simulink model "Lorenzo_comparison_simulation"  (R2023b)
settings: Solver=ode5  StartTime=0.0  StopTime=8  FixedStep=0.00005  RelTol=1e-3
settings Model: Creator=amaiani  LastModifiedBy=amaiani

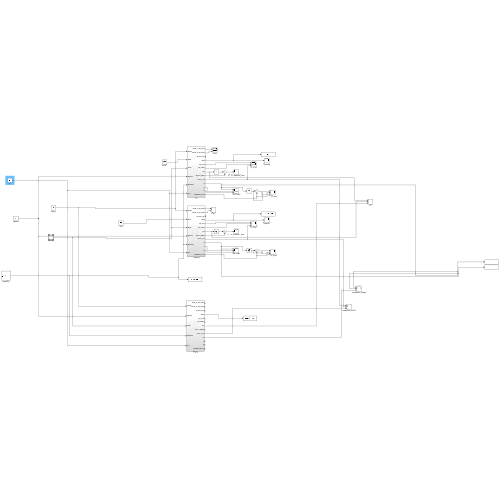
[thumbnail: Simulink's stored preview of the top-level diagram]
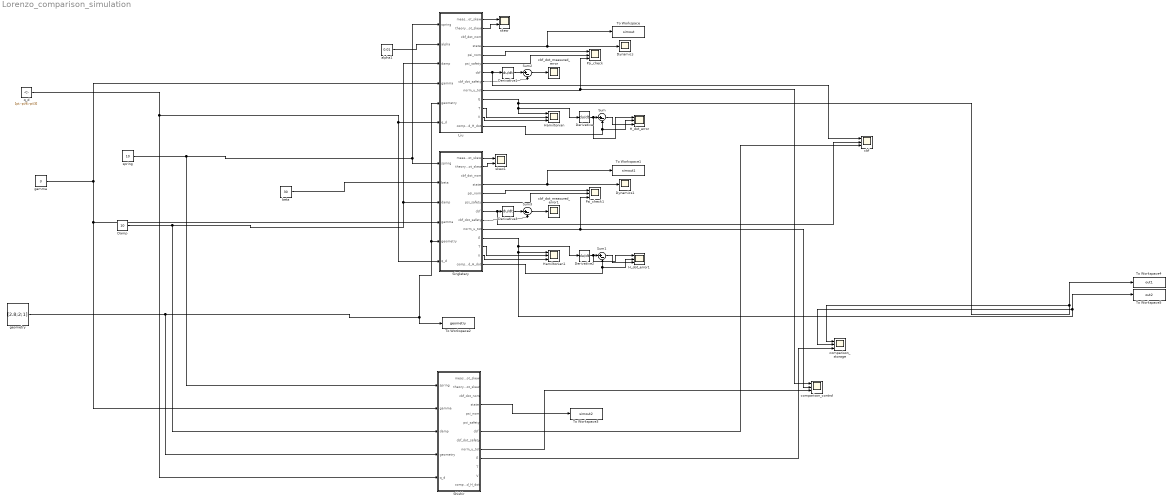
== system Lorenzo_comparison_simulation ==
  Damp : Constant  Value=10
  Derivative{,1..3} (4 alike) : Derivative
  Dynamics : Scope
  Dynamics1 : Scope
  H_dot_error : Scope  NumInputPorts=3
  H_dot_error1 : Scope  NumInputPorts=3
  Hamiltonian : Scope  NumInputPorts=3
  Hamiltonian1 : Scope  NumInputPorts=3
  Liu : Subsystem
  Psi_check : Scope  NumInputPorts=3
  Psi_check1 : Scope  NumInputPorts=3
  Shishir : Subsystem
  Singletary : Subsystem
  Sum{,1..3} (4 alike) : Sum  Inputs=|+-
  To Workspace : ToWorkspace  VariableName=simout  SampleTime=-1
  To Workspace1 : ToWorkspace  VariableName=simout1  SampleTime=-1
  To Workspace2 : ToWorkspace  VariableName=geometry  SampleTime=-1
  To Workspace3 : ToWorkspace  VariableName=simout2  SampleTime=-1
  To Workspace4 : ToWorkspace  VariableName=out1  SampleTime=-1
  To Workspace5 : ToWorkspace  VariableName=out2  SampleTime=-1
  alpha1 : Constant  Value=0.01
  beta : Constant  Value=30
  cbf : Scope  NumInputPorts=3
  cbf_dot_measured_error : Scope
  cbf_dot_measured_error1 : Scope
  comparison_control : Scope  NumInputPorts=3
  comparison_storage : Scope  NumInputPorts=3
  gamma : Constant  Value=3
  geometry : Constant  Value=[2.8;2;1]
  q_d : Constant  Value=[pi;-pi/6;-pi/3]
  skew : Scope  NumInputPorts=2
  skew1 : Scope  NumInputPorts=2
  spring : Constant  Value=10
  wires:
  Liu/10(E) -> To Workspace4/1, comparison_storage/1, Derivative/1, Hamiltonian/1
  Liu/1(meas_m_dot_skew) -> skew/1
  Liu/2(theory_m_dot_skew) -> skew/2
  Liu/13(computed_H_dot) -> H_dot_error/2, Sum/2
  Liu/7(cbf) -> cbf/1, Derivative1/1
  Derivative1/1 -> Sum2/1
  Sum2/1 -> cbf_dot_measured_error/1
  Liu/8(cbf_dot_safety) -> Sum2/2
  Liu/11(T) -> Hamiltonian/2
  Liu/12(V) -> Hamiltonian/3
  gamma/1 -> Singletary/4(gamma), Shishir/2(gamma), Liu/4(gamma)
  Derivative/1 -> H_dot_error/1, Sum/1
  Sum/1 -> H_dot_error/3
  Liu/9(norm_u_tot) -> comparison_control/1, Psi_check/3
  Liu/6(psi_safety) -> Psi_check/2
  Liu/5(psi_nom) -> Psi_check/1
  Liu/4(state) -> Dynamics/1, To Workspace/1
  Singletary/2(theory_m_dot_skew) -> skew1/2
  Sum3/1 -> cbf_dot_measured_error1/1
  Singletary/8(cbf_dot_safety) -> Sum3/2
  Singletary/11(T) -> Hamiltonian1/2
  Derivative3/1 -> Sum3/1
  Singletary/12(V) -> Hamiltonian1/3
  Singletary/4(state) -> Dynamics1/1, To Workspace1/1
  Singletary/6(psi_safety) -> Psi_check1/2
  Singletary/1(meas_m_dot_skew) -> skew1/1
  Singletary/5(psi_nom) -> Psi_check1/1
  Derivative2/1 -> H_dot_error1/1, Sum1/1
  Singletary/13(computed_H_dot) -> H_dot_error1/2, Sum1/2
  Singletary/9(norm_u_tot) -> comparison_control/2, Psi_check1/3
  Sum1/1 -> H_dot_error1/3
  Singletary/7(cbf) -> cbf/2, Derivative3/1
  geometry/1 -> Shishir/4(geometry), Liu/5(geometry), Singletary/5(geometry), To Workspace2/1
  alpha1/1 -> Liu/2(alpha)
  Damp/1 -> Shishir/3(damp), Singletary/3(damp), Liu/3(damp)
  spring/1 -> Shishir/1(spring), Singletary/1(spring), Liu/1(spring)
  beta/1 -> Singletary/2(beta)
  Singletary/10(E) -> To Workspace5/1, comparison_storage/2, Hamiltonian1/1, Derivative2/1
  Shishir/7(cbf) -> cbf/3
  Shishir/10(E) -> comparison_storage/3
  Shishir/9(norm_u_tot) -> comparison_control/3
  q_d/1 -> Shishir/5(q_d), Liu/6(q_d), Singletary/6(q_d)
  Shishir/4(state) -> To Workspace3/1

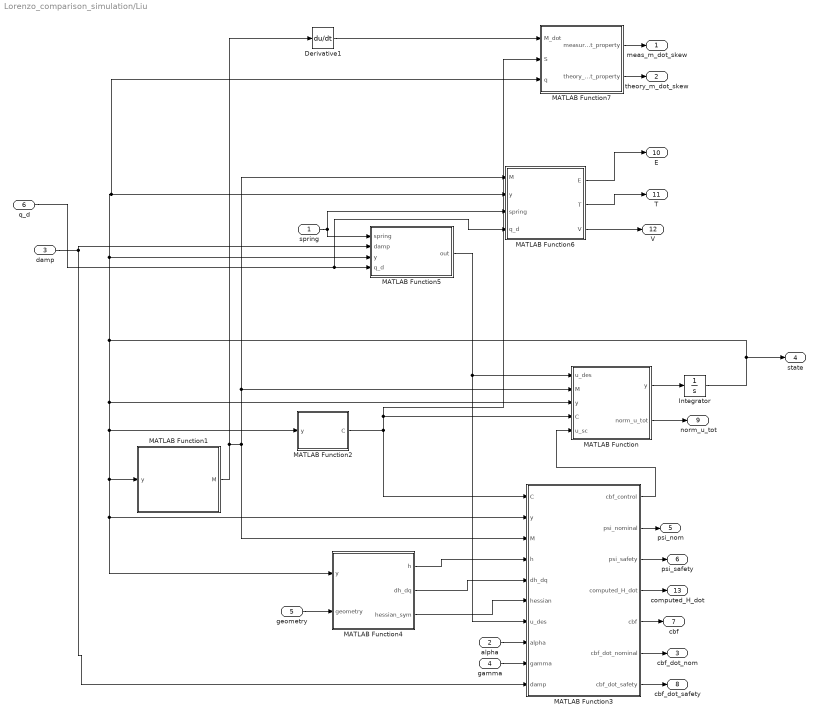
== system Lorenzo_comparison_simulation/Liu ==
  spring : Inport
  alpha : Inport  Port=2
  damp : Inport  Port=3
  gamma : Inport  Port=4
  geometry : Inport  Port=5
  q_d : Inport  Port=6
  Derivative1 : Derivative
  Integrator : Integrator  InitialCondition=[0;0;0;0;0;0]
  MATLAB Function : MATLAB Function  TreatAsAtomicUnit=on
  MATLAB Function1 : MATLAB Function  StartFcn=|  TreatAsAtomicUnit=on
      | % Define numerical values for the parameters
      | xc = 2.5;
      | yc = 2;
      | r = 1;
      | gamma = 2;
      | alpha = 20;
      | 
      | 
      | m1 = 1;
      | m2 = 1;
      | m3 = 1;
      | 
      | 
      | l1 = 1;
      | l2 = 1;
      | l3 = 1;
  MATLAB Function2 : MATLAB Function  StartFcn=|  TreatAsAtomicUnit=on
      | % Define numerical values for the parameters
      | xc = 2.5;
      | yc = 2;
      | r = 1;
      | gamma = 2;
      | alpha = 20;
      | 
      | 
      | m1 = 1;
      | m2 = 1;
      | m3 = 1;
      | 
      | 
      | l1 = 1;
      | l2 = 1;
      | l3 = 1;
  MATLAB Function3 : MATLAB Function  TreatAsAtomicUnit=on
  MATLAB Function4 : MATLAB Function  TreatAsAtomicUnit=on
  MATLAB Function5 : MATLAB Function  TreatAsAtomicUnit=on
  MATLAB Function6 : MATLAB Function  TreatAsAtomicUnit=on
  MATLAB Function7 : MATLAB Function  StartFcn=|  TreatAsAtomicUnit=on
      | % Define numerical values for the parameters
      | xc = 2.5;
      | yc = 2;
      | r = 1;
      | gamma = 2;
      | alpha = 20;
      | 
      | 
      | m1 = 1;
      | m2 = 1;
      | m3 = 1;
      | 
      | 
      | l1 = 1;
      | l2 = 1;
      | l3 = 1;
  meas_m_dot_skew : Outport
  theory_m_dot_skew : Outport  Port=2
  cbf_dot_nom : Outport  Port=3
  state : Outport  Port=4
  psi_nom : Outport  Port=5
  psi_safety : Outport  Port=6
  cbf : Outport  Port=7
  cbf_dot_safety : Outport  Port=8
  norm_u_tot : Outport  Port=9
  E : Outport  Port=10
  T : Outport  Port=11
  V : Outport  Port=12
  computed_H_dot : Outport  Port=13
  wires:
  MATLAB Function3/7(cbf_dot_safety) -> cbf_dot_safety/1
  MATLAB Function3/2(psi_nominal) -> psi_nom/1
  MATLAB Function3/5(cbf) -> cbf/1
  MATLAB Function/2(norm_u_tot) -> norm_u_tot/1
  MATLAB Function4/3(hessian_sym) -> MATLAB Function3/6(hessian)
  MATLAB Function1/1(M) -> Derivative1/1, MATLAB Function6/1(M), MATLAB Function/2(M), MATLAB Function3/3(M)
  MATLAB Function4/2(dh_dq) -> MATLAB Function3/5(dh_dq)
  MATLAB Function7/1(measured_m_dot_property) -> meas_m_dot_skew/1
  alpha/1 -> MATLAB Function3/8(alpha)
  MATLAB Function6/1(E) -> E/1
  MATLAB Function3/3(psi_safety) -> psi_safety/1
  MATLAB Function7/2(theory_m_dot_property) -> theory_m_dot_skew/1
  MATLAB Function3/4(computed_H_dot) -> computed_H_dot/1
  Derivative1/1 -> MATLAB Function7/1(M_dot)
  q_d/1 -> MATLAB Function6/4(q_d), MATLAB Function5/4(q_d)
  MATLAB Function3/6(cbf_dot_nominal) -> cbf_dot_nom/1
  MATLAB Function/1(y) -> Integrator/1
  MATLAB Function3/1(cbf_control) -> MATLAB Function/5(u_sc)
  MATLAB Function2/1(C) -> MATLAB Function/4(C), MATLAB Function7/2(S), MATLAB Function3/1(C)
  MATLAB Function4/1(h) -> MATLAB Function3/4(h)
  spring/1 -> MATLAB Function6/3(spring), MATLAB Function5/1(spring)
  MATLAB Function5/1(out) -> MATLAB Function3/7(u_des), MATLAB Function/1(u_des)
  Integrator/1 -> MATLAB Function7/3(q), MATLAB Function6/2(y), MATLAB Function5/3(y), MATLAB Function4/1(y), MATLAB Function3/2(y), MATLAB Function1/1(y), MATLAB Function2/1(y), MATLAB Function/3("y "), state/1
  damp/1 -> MATLAB Function3/10(damp), MATLAB Function5/2(damp)
  MATLAB Function6/2(T) -> T/1
  MATLAB Function6/3(V) -> V/1
  gamma/1 -> MATLAB Function3/9(gamma)
  geometry/1 -> MATLAB Function4/2(geometry)

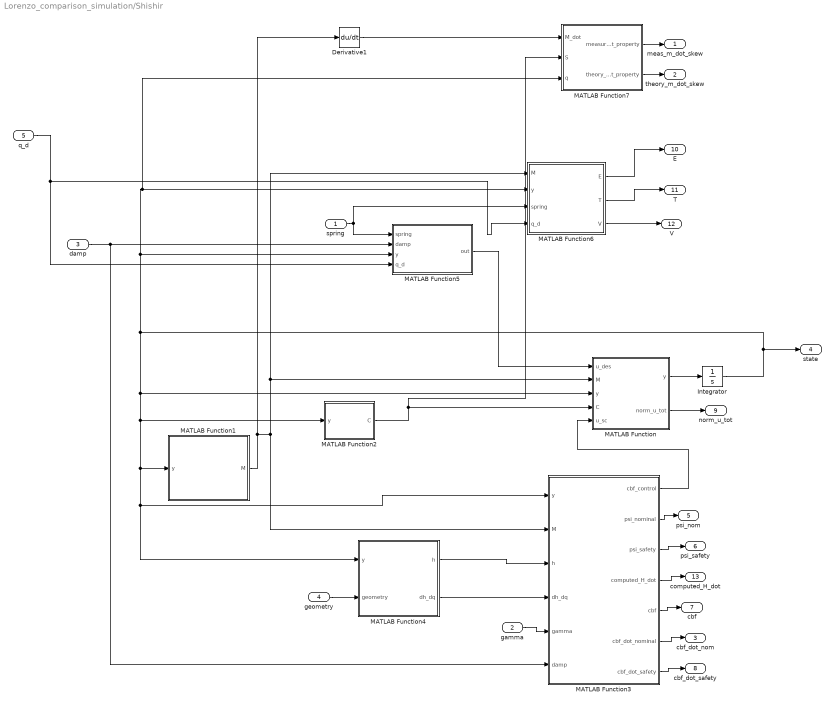
== system Lorenzo_comparison_simulation/Shishir ==
  spring : Inport
  gamma : Inport  Port=2
  damp : Inport  Port=3
  geometry : Inport  Port=4
  q_d : Inport  Port=5
  Derivative1 : Derivative
  Integrator : Integrator  InitialCondition=[0;0;0;0;0;0]
  MATLAB Function : MATLAB Function  TreatAsAtomicUnit=on
  MATLAB Function1 : MATLAB Function  StartFcn=|  TreatAsAtomicUnit=on
      | % Define numerical values for the parameters
      | xc = 2.5;
      | yc = 2;
      | r = 1;
      | gamma = 2;
      | alpha = 20;
      | 
      | 
      | m1 = 1;
      | m2 = 1;
      | m3 = 1;
      | 
      | 
      | l1 = 1;
      | l2 = 1;
      | l3 = 1;
  MATLAB Function2 : MATLAB Function  StartFcn=|  TreatAsAtomicUnit=on
      | % Define numerical values for the parameters
      | xc = 2.5;
      | yc = 2;
      | r = 1;
      | gamma = 2;
      | alpha = 20;
      | 
      | 
      | m1 = 1;
      | m2 = 1;
      | m3 = 1;
      | 
      | 
      | l1 = 1;
      | l2 = 1;
      | l3 = 1;
  MATLAB Function3 : MATLAB Function  TreatAsAtomicUnit=on
  MATLAB Function4 : MATLAB Function  TreatAsAtomicUnit=on
  MATLAB Function5 : MATLAB Function  TreatAsAtomicUnit=on
  MATLAB Function6 : MATLAB Function  TreatAsAtomicUnit=on
  MATLAB Function7 : MATLAB Function  StartFcn=|  TreatAsAtomicUnit=on
      | % Define numerical values for the parameters
      | xc = 2.5;
      | yc = 2;
      | r = 1;
      | gamma = 2;
      | alpha = 20;
      | 
      | 
      | m1 = 1;
      | m2 = 1;
      | m3 = 1;
      | 
      | 
      | l1 = 1;
      | l2 = 1;
      | l3 = 1;
  meas_m_dot_skew : Outport
  theory_m_dot_skew : Outport  Port=2
  cbf_dot_nom : Outport  Port=3
  state : Outport  Port=4
  psi_nom : Outport  Port=5
  psi_safety : Outport  Port=6
  cbf : Outport  Port=7
  cbf_dot_safety : Outport  Port=8
  norm_u_tot : Outport  Port=9
  E : Outport  Port=10
  T : Outport  Port=11
  V : Outport  Port=12
  computed_H_dot : Outport  Port=13
  wires:
  MATLAB Function3/7(cbf_dot_safety) -> cbf_dot_safety/1
  MATLAB Function3/2(psi_nominal) -> psi_nom/1
  MATLAB Function3/5(cbf) -> cbf/1
  MATLAB Function/2(norm_u_tot) -> norm_u_tot/1
  MATLAB Function1/1(M) -> Derivative1/1, MATLAB Function6/1(M), MATLAB Function/2(M), MATLAB Function3/2(M)
  MATLAB Function4/2(dh_dq) -> MATLAB Function3/4(dh_dq)
  MATLAB Function7/1(measured_m_dot_property) -> meas_m_dot_skew/1
  gamma/1 -> MATLAB Function3/5(gamma)
  MATLAB Function6/1(E) -> E/1
  MATLAB Function3/3(psi_safety) -> psi_safety/1
  MATLAB Function7/2(theory_m_dot_property) -> theory_m_dot_skew/1
  MATLAB Function3/4(computed_H_dot) -> computed_H_dot/1
  Derivative1/1 -> MATLAB Function7/1(M_dot)
  q_d/1 -> MATLAB Function6/4(q_d), MATLAB Function5/4(q_d)
  MATLAB Function3/6(cbf_dot_nominal) -> cbf_dot_nom/1
  MATLAB Function/1(y) -> Integrator/1
  MATLAB Function3/1(cbf_control) -> MATLAB Function/5(u_sc)
  MATLAB Function2/1(C) -> MATLAB Function/4(C), MATLAB Function7/2(S)
  MATLAB Function4/1(h) -> MATLAB Function3/3(h)
  spring/1 -> MATLAB Function6/3(spring), MATLAB Function5/1(spring)
  MATLAB Function5/1(out) -> MATLAB Function/1(u_des)
  Integrator/1 -> MATLAB Function7/3(q), MATLAB Function6/2(y), MATLAB Function5/3(y), MATLAB Function4/1(y), MATLAB Function3/1(y), MATLAB Function1/1(y), MATLAB Function2/1(y), MATLAB Function/3("y "), state/1
  damp/1 -> MATLAB Function3/6(damp), MATLAB Function5/2(damp)
  MATLAB Function6/2(T) -> T/1
  MATLAB Function6/3(V) -> V/1
  geometry/1 -> MATLAB Function4/2(geometry)

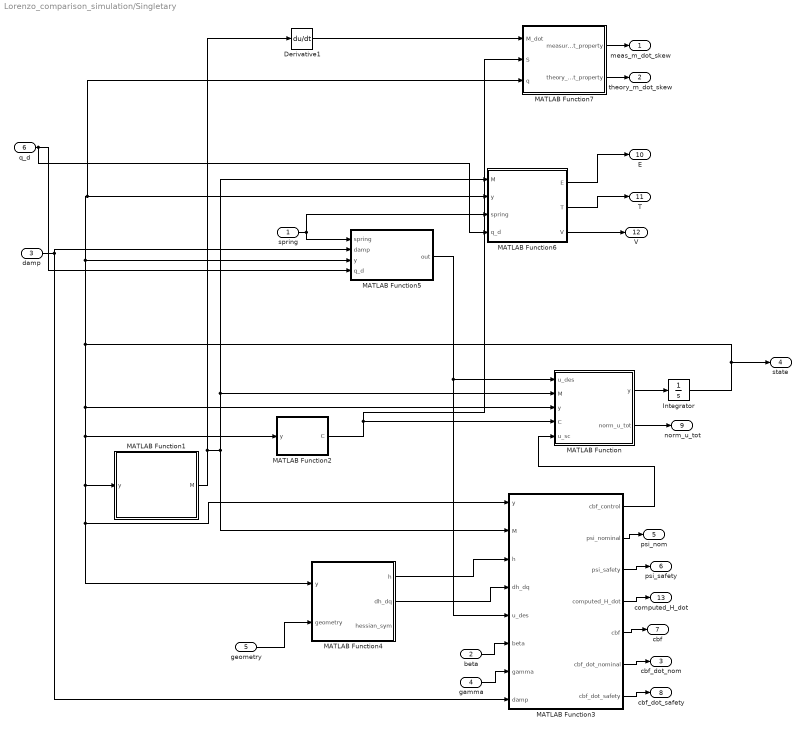
== system Lorenzo_comparison_simulation/Singletary ==
  spring : Inport
  beta : Inport  Port=2
  damp : Inport  Port=3
  gamma : Inport  Port=4
  geometry : Inport  Port=5
  q_d : Inport  Port=6
  Derivative1 : Derivative
  Integrator : Integrator  InitialCondition=[0;0;0;0;0;0]
  MATLAB Function : MATLAB Function  TreatAsAtomicUnit=on
  MATLAB Function1 : MATLAB Function  StartFcn=|  TreatAsAtomicUnit=on
      | % Define numerical values for the parameters
      | xc = 2.5;
      | yc = 2;
      | r = 1;
      | gamma = 2;
      | alpha = 20;
      | 
      | 
      | m1 = 1;
      | m2 = 1;
      | m3 = 1;
      | 
      | 
      | l1 = 1;
      | l2 = 1;
      | l3 = 1;
  MATLAB Function2 : MATLAB Function  StartFcn=|  TreatAsAtomicUnit=on
      | % Define numerical values for the parameters
      | xc = 2.5;
      | yc = 2;
      | r = 1;
      | gamma = 2;
      | alpha = 20;
      | 
      | 
      | m1 = 1;
      | m2 = 1;
      | m3 = 1;
      | 
      | 
      | l1 = 1;
      | l2 = 1;
      | l3 = 1;
  MATLAB Function3 : MATLAB Function  TreatAsAtomicUnit=on
  MATLAB Function4 : MATLAB Function  TreatAsAtomicUnit=on
  MATLAB Function5 : MATLAB Function  TreatAsAtomicUnit=on
  MATLAB Function6 : MATLAB Function  TreatAsAtomicUnit=on
  MATLAB Function7 : MATLAB Function  StartFcn=|  TreatAsAtomicUnit=on
      | % Define numerical values for the parameters
      | xc = 2.5;
      | yc = 2;
      | r = 1;
      | gamma = 2;
      | alpha = 20;
      | 
      | 
      | m1 = 1;
      | m2 = 1;
      | m3 = 1;
      | 
      | 
      | l1 = 1;
      | l2 = 1;
      | l3 = 1;
  meas_m_dot_skew : Outport
  theory_m_dot_skew : Outport  Port=2
  cbf_dot_nom : Outport  Port=3
  state : Outport  Port=4
  psi_nom : Outport  Port=5
  psi_safety : Outport  Port=6
  cbf : Outport  Port=7
  cbf_dot_safety : Outport  Port=8
  norm_u_tot : Outport  Port=9
  E : Outport  Port=10
  T : Outport  Port=11
  V : Outport  Port=12
  computed_H_dot : Outport  Port=13
  wires:
  MATLAB Function3/7(cbf_dot_safety) -> cbf_dot_safety/1
  MATLAB Function3/2(psi_nominal) -> psi_nom/1
  MATLAB Function3/5(cbf) -> cbf/1
  MATLAB Function/2(norm_u_tot) -> norm_u_tot/1
  MATLAB Function1/1(M) -> Derivative1/1, MATLAB Function6/1(M), MATLAB Function/2(M), MATLAB Function3/2(M)
  MATLAB Function4/2(dh_dq) -> MATLAB Function3/4(dh_dq)
  MATLAB Function7/1(measured_m_dot_property) -> meas_m_dot_skew/1
  beta/1 -> MATLAB Function3/6(beta)
  MATLAB Function6/1(E) -> E/1
  MATLAB Function3/3(psi_safety) -> psi_safety/1
  MATLAB Function7/2(theory_m_dot_property) -> theory_m_dot_skew/1
  MATLAB Function3/4(computed_H_dot) -> computed_H_dot/1
  Derivative1/1 -> MATLAB Function7/1(M_dot)
  q_d/1 -> MATLAB Function6/4(q_d), MATLAB Function5/4(q_d)
  MATLAB Function3/6(cbf_dot_nominal) -> cbf_dot_nom/1
  MATLAB Function/1(y) -> Integrator/1
  MATLAB Function3/1(cbf_control) -> MATLAB Function/5(u_sc)
  MATLAB Function2/1(C) -> MATLAB Function/4(C), MATLAB Function7/2(S)
  MATLAB Function4/1(h) -> MATLAB Function3/3(h)
  spring/1 -> MATLAB Function6/3(spring), MATLAB Function5/1(spring)
  MATLAB Function5/1(out) -> MATLAB Function3/5(u_des), MATLAB Function/1(u_des)
  Integrator/1 -> MATLAB Function7/3(q), MATLAB Function6/2(y), MATLAB Function5/3(y), MATLAB Function4/1(y), MATLAB Function3/1(y), MATLAB Function1/1(y), MATLAB Function2/1(y), MATLAB Function/3("y "), state/1
  damp/1 -> MATLAB Function3/8(damp), MATLAB Function5/2(damp)
  MATLAB Function6/2(T) -> T/1
  MATLAB Function6/3(V) -> V/1
  gamma/1 -> MATLAB Function3/7(gamma)
  geometry/1 -> MATLAB Function4/2(geometry)

== matlab function Lorenzo_comparison_simulation/Liu/MATLAB Function7 ==
  data: M_dot input; measured_m_dot_property output; S input; q input; theory_m_dot_property output


function [measured_m_dot_property, theory_m_dot_property] = M_dot_coriolis_check(M_dot,S, q)
    dq = reshape(q(4:6),[3,1]);
    
    q1 = q(1);
    q2 = q(2);
    q3 = q(3);
    dq1 = q(4);
    dq2 = q(5);
    dq3 = q(6);

    check = M_dot - 2 * S;


    measured_m_dot_property = dq' * check * dq;


    M_dot_formula =   [        - dq2*(sin(q2 + q3) + 3*sin(q2)) - dq3*(sin(q2 + q3) + sin(q3)), - dq3*(sin(q2 + q3)/2 + sin(q3)) - dq2*(sin(q2 + q3)/2 + (3*sin(q2))/2), - (dq2*sin(q2 + q3))/2 - dq3*(sin(q2 + q3)/2 + sin(q3)/2);
- dq3*(sin(q2 + q3)/2 + sin(q3)) - dq2*(sin(q2 + q3)/2 + (3*sin(q2))/2),                                                            -dq3*sin(q3),                                          -(dq3*sin(q3))/2;
              - (dq2*sin(q2 + q3))/2 - dq3*(sin(q2 + q3)/2 + sin(q3)/2),                                                        -(dq3*sin(q3))/2,                                                         0];
 

    
    theory_m_dot_property = dq' * (M_dot_formula - 2 * S) * dq;
end

== matlab function Lorenzo_comparison_simulation/Singletary/MATLAB Function ==
  data: u_des input; M input; y input; y output; C input; u_sc input; norm_u_tot output
function [y,norm_u_tot]= dynamics(u_des, M,y, C, u_sc)
    
    q = reshape(y(1:3),[3,1]);
    dq = reshape(y(4:6),[3,1]);



    [~, p] = chol(M);
    decision = (p == 0);

    assert(decision, 'Inertia matrix is not positive definite');
    
    u_tot = u_des + u_sc;
    norm_u_tot=norm(u_tot);
    ddq = inv(M) * (u_tot - C * dq ); 

    y = [dq; ddq];

== matlab function Lorenzo_comparison_simulation/Singletary/MATLAB Function1 ==
  data: y input; M output
function M = inertia_M(y)

    q1 = y(1);
    q2 = y(2);
    q3 = y(3);

    M  = [        cos(q2 + q3) + 3*cos(q2) + cos(q3) + 4, cos(q2 + q3)/2 + (3*cos(q2))/2 + cos(q3) + 5/3, cos(q2 + q3)/2 + cos(q3)/2 + 1/3;
cos(q2 + q3)/2 + (3*cos(q2))/2 + cos(q3) + 5/3,                                  cos(q3) + 5/3,                  cos(q3)/2 + 1/3;
              cos(q2 + q3)/2 + cos(q3)/2 + 1/3,                                cos(q3)/2 + 1/3,                              1/3];

    assert(isequal(M, M'),'error')

== matlab function Lorenzo_comparison_simulation/Singletary/MATLAB Function2 ==
  data: y input; C output
function C = coriolis(y)

    q1 = y(1);
    q2 = y(2);
    q3 = y(3);
    dq1 = y(4);
    dq2 = y(5);
    dq3 = y(6);


    C = [- dq2*(sin(q2 + q3)/2 + (3*sin(q2))/2) - dq3*(sin(q2 + q3)/2 + sin(q3)/2), - dq1*(sin(q2 + q3)/2 + (3*sin(q2))/2) - dq2*(sin(q2 + q3)/2 + (3*sin(q2))/2) - dq3*(sin(q2 + q3)/2 + sin(q3)/2), - dq1*(sin(q2 + q3)/2 + sin(q3)/2) - dq2*(sin(q2 + q3)/2 + sin(q3)/2) - dq3*(sin(q2 + q3)/2 + sin(q3)/2);
                dq1*(sin(q2 + q3)/2 + (3*sin(q2))/2) - (dq3*sin(q3))/2,                                                                                                 -(dq3*sin(q3))/2,                                                    - (dq1*sin(q3))/2 - (dq2*sin(q3))/2 - (dq3*sin(q3))/2;
                       dq1*(sin(q2 + q3)/2 + sin(q3)/2) + (dq2*sin(q3))/2,                                                                                (dq1*sin(q3))/2 + (dq2*sin(q3))/2,                                                                                                        0];

== matlab function Lorenzo_comparison_simulation/Singletary/MATLAB Function3 ==
  data: y input; cbf_control output; M input; h input; dh_dq input; u_des input; psi_nominal output; psi_safety output; computed_H_dot output; cbf output; cbf_dot_nominal output; cbf_dot_safety output; beta input; gamma input; damp input
function [cbf_control, psi_nominal, psi_safety, computed_H_dot, cbf, cbf_dot_nominal,cbf_dot_safety]= CBF(y, M, h, dh_dq, u_des, beta, gamma, damp)
    
    q = reshape(y(1:3),[3,1]);
    dq = reshape(y(4:6),[3,1]);
    dh_dq = reshape(dh_dq,[1,3]);

    M_inv = inv(M);


    KE = 0.5 * dq' * M * dq;
    cbf = beta * h - KE;

    cbf_dot_nominal = dq' * (beta .* dh_dq'- u_des);
    psi_nominal = cbf_dot_nominal + gamma .* cbf;
    if psi_nominal<0
        lg_h = -dq';
        cbf_control =  -lg_h' /(lg_h * lg_h')  .* psi_nominal;
    else
        cbf_control = zeros(3,1);
    end
    cbf_dot_safety =  dq' * (beta .* dh_dq'- u_des- cbf_control);
    psi_safety = cbf_dot_safety + gamma .* cbf;

    computed_H_dot = dq' * cbf_control - dq' * damp * dq;
end

== matlab function Lorenzo_comparison_simulation/Singletary/MATLAB Function4 ==
  data: y input; h output; dh_dq output; hessian_sym output; geometry input
function [h, dh_dq, hessian_sym] = obstacle(y, geometry)
    % Define numerical values for the parameters
    % xc = 2.5;
    % yc = 2;
    % r = 1;
    xc = geometry(1);
    yc = geometry(2);
    r = geometry(3);

    l1 = 1;
    l2 = 1;
    l3 = 1;
    
    % Compute the end-effector position using forward kinematics
    q1 = y(1);
    q2 = y(2);
    q3 = y(3);
    
    x_ee = l1 * cos(q1) + l2 * cos(q1 + q2) + l3 * cos(q1 + q2 + q3);
    y_ee = l1 * sin(q1) + l2 * sin(q1 + q2) + l3 * sin(q1 + q2 + q3);
    
    % Compute the control barrier function h
    h = (xc - x_ee)^2 + (yc - y_ee)^2 - r^2;
    
    % Define the expressions for dh_dq and hessian_sym
    dh_dq = [2*(cos(q1 + q2 + q3) + cos(q1 + q2) + cos(q1))*(sin(q1 + q2 + q3) + sin(q1 + q2) + sin(q1) - 2) - 2*(sin(q1 + q2 + q3) + sin(q1 + q2) + sin(q1))*(cos(q1 + q2 + q3) + cos(q1 + q2) + cos(q1) - 5/2), 2*(cos(q1 + q2 + q3) + cos(q1 + q2))*(sin(q1 + q2 + q3) + sin(q1 + q2) + sin(q1) - 2) - 2*(sin(q1 + q2 + q3) + sin(q1 + q2))*(cos(q1 + q2 + q3) + cos(q1 + q2) + cos(q1) - 5/2), 2*cos(q1 + q2 + q3)*(sin(q1 + q2 + q3) + sin(q1 + q2) + sin(q1) - 2) - 2*sin(q1 + q2 + q3)*(cos(q1 + q2 + q3) + cos(q1 + q2) + cos(q1) - 5/2)];


    hessian_sym = [                                              2*(cos(q1 + q2 + q3) + cos(q1 + q2) + cos(q1))^2 - 2*(cos(q1 + q2 + q3) + cos(q1 + q2) + cos(q1))*(cos(q1 + q2 + q3) + cos(q1 + q2) + cos(q1) - 5/2) + 2*(sin(q1 + q2 + q3) + sin(q1 + q2) + sin(q1))^2 - 2*(sin(q1 + q2 + q3) + sin(q1 + q2) + sin(q1))*(sin(q1 + q2 + q3) + sin(q1 + q2) + sin(q1) - 2), 2*(cos(q1 + q2 + q3) + cos(q1 + q2))*(cos(q1 + q2 + q3) + cos(q1 + q2) + cos(q1)) - 2*(cos(q1 + q2 + q3) + cos(q1 + q2))*(cos(q1 + q2 + q3) + cos(q1 + q2) + cos(q1) - 5/2) + 2*(sin(q1 + q2 + q3) + sin(q1 + q2))*(sin(q1 + q2 + q3) + sin(q1 + q2) + sin(q1)) - 2*(sin(q1 + q2 + q3) + sin(q1 + q2))*(sin(q1 + q2 + q3) + sin(q1 + q2) + sin(q1) - 2), 2*cos(q1 + q2 + q3)*(cos(q1 + q2 + q3) + cos(q1 + q2) + cos(q1)) - 2*cos(q1 + q2 + q3)*(cos(q1 + q2 + q3) + cos(q1 + q2) + cos(q1) - 5/2) + 2*sin(q1 + q2 + q3)*(sin(q1 + q2 + q3) + sin(q1 + q2) + sin(q1)) - 2*sin(q1 + q2 + q3)*(sin(q1 + q2 + q3) + sin(q1 + q2) + sin(q1) - 2);
        2*(cos(q1 + q2 + q3) + cos(q1 + q2))*(cos(q1 + q2 + q3) + cos(q1 + q2) + cos(q1)) - 2*(cos(q1 + q2 + q3) + cos(q1 + q2))*(cos(q1 + q2 + q3) + cos(q1 + q2) + cos(q1) - 5/2) + 2*(sin(q1 + q2 + q3) + sin(q1 + q2))*(sin(q1 + q2 + q3) + sin(q1 + q2) + sin(q1)) - 2*(sin(q1 + q2 + q3) + sin(q1 + q2))*(sin(q1 + q2 + q3) + sin(q1 + q2) + sin(q1) - 2),                                                                                       2*(cos(q1 + q2 + q3) + cos(q1 + q2))^2 - 2*(cos(q1 + q2 + q3) + cos(q1 + q2))*(cos(q1 + q2 + q3) + cos(q1 + q2) + cos(q1) - 5/2) + 2*(sin(q1 + q2 + q3) + sin(q1 + q2))^2 - 2*(sin(q1 + q2 + q3) + sin(q1 + q2))*(sin(q1 + q2 + q3) + sin(q1 + q2) + sin(q1) - 2),                     2*cos(q1 + q2 + q3)*(cos(q1 + q2 + q3) + cos(q1 + q2)) - 2*cos(q1 + q2 + q3)*(cos(q1 + q2 + q3) + cos(q1 + q2) + cos(q1) - 5/2) - 2*sin(q1 + q2 + q3)*(sin(q1 + q2 + q3) + sin(q1 + q2) + sin(q1) - 2) + 2*sin(q1 + q2 + q3)*(sin(q1 + q2 + q3) + sin(q1 + q2));
                                                                            2*cos(q1 + q2 + q3)*(cos(q1 + q2 + q3) + cos(q1 + q2) + cos(q1)) - 2*cos(q1 + q2 + q3)*(cos(q1 + q2 + q3) + cos(q1 + q2) + cos(q1) - 5/2) + 2*sin(q1 + q2 + q3)*(sin(q1 + q2 + q3) + sin(q1 + q2) + sin(q1)) - 2*sin(q1 + q2 + q3)*(sin(q1 + q2 + q3) + sin(q1 + q2) + sin(q1) - 2),                                                                                         2*cos(q1 + q2 + q3)*(cos(q1 + q2 + q3) + cos(q1 + q2)) - 2*cos(q1 + q2 + q3)*(cos(q1 + q2 + q3) + cos(q1 + q2) + cos(q1) - 5/2) - 2*sin(q1 + q2 + q3)*(sin(q1 + q2 + q3) + sin(q1 + q2) + sin(q1) - 2) + 2*sin(q1 + q2 + q3)*(sin(q1 + q2 + q3) + sin(q1 + q2)),                                                                                       2*cos(q1 + q2 + q3)^2 - 2*cos(q1 + q2 + q3)*(cos(q1 + q2 + q3) + cos(q1 + q2) + cos(q1) - 5/2) + 2*sin(q1 + q2 + q3)^2 - 2*sin(q1 + q2 + q3)*(sin(q1 + q2 + q3) + sin(q1 + q2) + sin(q1) - 2)];
     

    % d = eig(hessian_sym)
    % isposdef = all(d >= 0);
    % 
    % assert(isposdef, 'error hessian');
end

== matlab function Lorenzo_comparison_simulation/Singletary/MATLAB Function5 ==
  data: spring input; damp input; y input; out output; q_d input
function out = u_des( spring, damp, y,q_d)


    q = reshape(y(1:3),[3,1]);
    dq = reshape(y(4:6),[3,1]);

    
    
    out =  - damp * dq - spring * (q-q_d);

== matlab function Lorenzo_comparison_simulation/Singletary/MATLAB Function6 ==
  data: M input; E output; y input; spring input; q_d input; T output; V output
function [E,T,V] = energy(M,y,spring, q_d)
    q = y(1:3);
    dq = y(4:6);
    
    T = 0.5 * (dq' * M * dq) ;
    V =0.5 * spring *(q-q_d)' * (q-q_d);
    E = T + V;

== matlab function Lorenzo_comparison_simulation/Singletary/MATLAB Function7 ==
  data: M_dot input; measured_m_dot_property output; S input; q input; theory_m_dot_property output


function [measured_m_dot_property, theory_m_dot_property] = M_dot_coriolis_check(M_dot,S, q)
    dq = reshape(q(4:6),[3,1]);
    
    q1 = q(1);
    q2 = q(2);
    q3 = q(3);
    dq1 = q(4);
    dq2 = q(5);
    dq3 = q(6);

    check = M_dot - 2 * S;


    measured_m_dot_property = dq' * check * dq;


    M_dot_formula =   [        - dq2*(sin(q2 + q3) + 3*sin(q2)) - dq3*(sin(q2 + q3) + sin(q3)), - dq3*(sin(q2 + q3)/2 + sin(q3)) - dq2*(sin(q2 + q3)/2 + (3*sin(q2))/2), - (dq2*sin(q2 + q3))/2 - dq3*(sin(q2 + q3)/2 + sin(q3)/2);
- dq3*(sin(q2 + q3)/2 + sin(q3)) - dq2*(sin(q2 + q3)/2 + (3*sin(q2))/2),                                                            -dq3*sin(q3),                                          -(dq3*sin(q3))/2;
              - (dq2*sin(q2 + q3))/2 - dq3*(sin(q2 + q3)/2 + sin(q3)/2),                                                        -(dq3*sin(q3))/2,                                                         0];
 

    
    theory_m_dot_property = dq' * (M_dot_formula - 2 * S) * dq;
end

== matlab function Lorenzo_comparison_simulation/Shishir/MATLAB Function ==
  data: u_des input; M input; y input; y output; C input; u_sc input; norm_u_tot output
function [y,norm_u_tot]= dynamics(u_des, M,y, C, u_sc)
    
    q = reshape(y(1:3),[3,1]);
    dq = reshape(y(4:6),[3,1]);



    [~, p] = chol(M);
    decision = (p == 0);

    assert(decision, 'Inertia matrix is not positive definite');
    
    u_tot = u_des + u_sc;
    norm_u_tot=norm(u_tot);
    ddq = inv(M) * (u_tot - C * dq ); 

    y = [dq; ddq];

== matlab function Lorenzo_comparison_simulation/Shishir/MATLAB Function1 ==
  data: y input; M output
function M = inertia_M(y)

    q1 = y(1);
    q2 = y(2);
    q3 = y(3);

    M  = [        cos(q2 + q3) + 3*cos(q2) + cos(q3) + 4, cos(q2 + q3)/2 + (3*cos(q2))/2 + cos(q3) + 5/3, cos(q2 + q3)/2 + cos(q3)/2 + 1/3;
cos(q2 + q3)/2 + (3*cos(q2))/2 + cos(q3) + 5/3,                                  cos(q3) + 5/3,                  cos(q3)/2 + 1/3;
              cos(q2 + q3)/2 + cos(q3)/2 + 1/3,                                cos(q3)/2 + 1/3,                              1/3];

    assert(isequal(M, M'),'error')

== matlab function Lorenzo_comparison_simulation/Shishir/MATLAB Function2 ==
  data: y input; C output
function C = coriolis(y)

    q1 = y(1);
    q2 = y(2);
    q3 = y(3);
    dq1 = y(4);
    dq2 = y(5);
    dq3 = y(6);


    C = [- dq2*(sin(q2 + q3)/2 + (3*sin(q2))/2) - dq3*(sin(q2 + q3)/2 + sin(q3)/2), - dq1*(sin(q2 + q3)/2 + (3*sin(q2))/2) - dq2*(sin(q2 + q3)/2 + (3*sin(q2))/2) - dq3*(sin(q2 + q3)/2 + sin(q3)/2), - dq1*(sin(q2 + q3)/2 + sin(q3)/2) - dq2*(sin(q2 + q3)/2 + sin(q3)/2) - dq3*(sin(q2 + q3)/2 + sin(q3)/2);
                dq1*(sin(q2 + q3)/2 + (3*sin(q2))/2) - (dq3*sin(q3))/2,                                                                                                 -(dq3*sin(q3))/2,                                                    - (dq1*sin(q3))/2 - (dq2*sin(q3))/2 - (dq3*sin(q3))/2;
                       dq1*(sin(q2 + q3)/2 + sin(q3)/2) + (dq2*sin(q3))/2,                                                                                (dq1*sin(q3))/2 + (dq2*sin(q3))/2,                                                                                                        0];

== matlab function Lorenzo_comparison_simulation/Shishir/MATLAB Function3 ==
  data: y input; cbf_control output; M input; h input; dh_dq input; psi_nominal output; psi_safety output; computed_H_dot output; cbf output; cbf_dot_nominal output; cbf_dot_safety output; gamma input; damp input
% 
% function [cbf_control, psi_nominal, psi_safety, computed_H_dot, cbf, cbf_dot_nominal,cbf_dot_safety]= CBF(C, y, M, h, dh_dq, hessian, u_des, alpha, gamma, damp)
% 
%     q = reshape(y(1:3),[3,1]);
%     dq = reshape(y(4:6),[3,1]);
%     dh_dq = reshape(dh_dq,[1,3]);
% 
%     M_inv = inv(M);
% 
%     cbf =  h + alpha * dh_dq * dq;
% 
%     cbf_dot_nominal =  dh_dq * dq + alpha * dq' * hessian * dq + alpha * dh_dq * (M_inv* (-C * dq + u_des));
%     psi_nominal = cbf_dot_nominal + gamma .* cbf;
%     if psi_nominal<0
%         lg_h = alpha * dh_dq * M_inv;
%         cbf_control =  - lg_h' /(lg_h * lg_h')  .* psi_nominal;
%     else
%         cbf_control = zeros(3,1);
%     end
%     cbf_dot_safety = dh_dq * dq + alpha * dq' * hessian * dq + alpha * dh_dq * (M_inv* (-C * dq + u_des + cbf_control));
%     psi_safety = cbf_dot_safety + gamma .* cbf;
% 
%     computed_H_dot = dq' * cbf_control - dq' * damp * dq;
% 
% end




function [cbf_control, psi_nominal, psi_safety, computed_H_dot, cbf, cbf_dot_nominal,cbf_dot_safety]= CBF(y, M, h, dh_dq, gamma, damp)

    q = reshape(y(1:3),[3,1]);
    dq = reshape(y(4:6),[3,1]);
    dh_dq = reshape(dh_dq,[1,3]);


    KE = 0.5 * dq' * M * dq;
    cbf = 1/h + KE/(1+KE);
    lg_h = dq'/(1+KE)^2;
    cbf_dot_nominal = - 1/h^2 * (dh_dq * dq)- 1/(1+KE)^2 * dq' * damp * dq;
    psi_nominal = cbf_dot_nominal - gamma .* h;
    if psi_nominal>0

        cbf_control =  -lg_h' /(lg_h*lg_h')  .* psi_nominal;
    else
        cbf_control = zeros(3,1);
    end
    cbf_dot_safety =  - 1/h^2 * (dh_dq * dq)- 1/(1+KE)^2 * dq' * damp * dq + lg_h * cbf_control;
    psi_safety = cbf_dot_safety - gamma .* h;

    computed_H_dot = dq' * cbf_control - dq' * damp * dq;

end

== matlab function Lorenzo_comparison_simulation/Shishir/MATLAB Function4 ==
  data: y input; h output; dh_dq output; geometry input
function [h, dh_dq] = obstacle(y, geometry)
    % Define numerical values for the parameters
    % xc = 2.5;
    % yc = 2;
    % r = 1;

    xc = geometry(1);
    yc = geometry(2);
    r = geometry(3);

    l1 = 1;
    l2 = 1;
    l3 = 1;
    
    % Compute the end-effector position using forward kinematics
    q1 = y(1);
    q2 = y(2);
    q3 = y(3);
    
    x_ee = l1 * cos(q1) + l2 * cos(q1 + q2) + l3 * cos(q1 + q2 + q3);
    y_ee = l1 * sin(q1) + l2 * sin(q1 + q2) + l3 * sin(q1 + q2 + q3);
    
    % Compute the control barrier function h
    h = (xc - x_ee)^2 + (yc - y_ee)^2 - r^2;
    
    % Define the expressions for dh_dq and hessian_sym
    dh_dq = [2*(cos(q1 + q2 + q3) + cos(q1 + q2) + cos(q1))*(sin(q1 + q2 + q3) + sin(q1 + q2) + sin(q1) - 2) - 2*(sin(q1 + q2 + q3) + sin(q1 + q2) + sin(q1))*(cos(q1 + q2 + q3) + cos(q1 + q2) + cos(q1) - 5/2), 2*(cos(q1 + q2 + q3) + cos(q1 + q2))*(sin(q1 + q2 + q3) + sin(q1 + q2) + sin(q1) - 2) - 2*(sin(q1 + q2 + q3) + sin(q1 + q2))*(cos(q1 + q2 + q3) + cos(q1 + q2) + cos(q1) - 5/2), 2*cos(q1 + q2 + q3)*(sin(q1 + q2 + q3) + sin(q1 + q2) + sin(q1) - 2) - 2*sin(q1 + q2 + q3)*(cos(q1 + q2 + q3) + cos(q1 + q2) + cos(q1) - 5/2)];

end

== matlab function Lorenzo_comparison_simulation/Shishir/MATLAB Function5 ==
  data: spring input; damp input; y input; out output; q_d input
function out = u_des( spring, damp, y,q_d)


    q = reshape(y(1:3),[3,1]);
    dq = reshape(y(4:6),[3,1]);

    
    
    out =  - damp * dq - spring * (q-q_d);

== matlab function Lorenzo_comparison_simulation/Shishir/MATLAB Function6 ==
  data: M input; E output; y input; spring input; q_d input; T output; V output
function [E,T,V] = energy(M,y,spring, q_d)
    q = y(1:3);
    dq = y(4:6);
    
    T = 0.5 * (dq' * M * dq) ;
    V =0.5 * spring *(q-q_d)' * (q-q_d);
    E = T + V;

== matlab function Lorenzo_comparison_simulation/Shishir/MATLAB Function7 ==
  data: M_dot input; measured_m_dot_property output; S input; q input; theory_m_dot_property output


function [measured_m_dot_property, theory_m_dot_property] = M_dot_coriolis_check(M_dot,S, q)
    dq = reshape(q(4:6),[3,1]);
    
    q1 = q(1);
    q2 = q(2);
    q3 = q(3);
    dq1 = q(4);
    dq2 = q(5);
    dq3 = q(6);

    check = M_dot - 2 * S;


    measured_m_dot_property = dq' * check * dq;


    M_dot_formula =   [        - dq2*(sin(q2 + q3) + 3*sin(q2)) - dq3*(sin(q2 + q3) + sin(q3)), - dq3*(sin(q2 + q3)/2 + sin(q3)) - dq2*(sin(q2 + q3)/2 + (3*sin(q2))/2), - (dq2*sin(q2 + q3))/2 - dq3*(sin(q2 + q3)/2 + sin(q3)/2);
- dq3*(sin(q2 + q3)/2 + sin(q3)) - dq2*(sin(q2 + q3)/2 + (3*sin(q2))/2),                                                            -dq3*sin(q3),                                          -(dq3*sin(q3))/2;
              - (dq2*sin(q2 + q3))/2 - dq3*(sin(q2 + q3)/2 + sin(q3)/2),                                                        -(dq3*sin(q3))/2,                                                         0];
 

    
    theory_m_dot_property = dq' * (M_dot_formula - 2 * S) * dq;
end

== matlab function Lorenzo_comparison_simulation/Liu/MATLAB Function1 ==
  data: y input; M output
function M = inertia_M(y)

    q1 = y(1);
    q2 = y(2);
    q3 = y(3);

    M  = [        cos(q2 + q3) + 3*cos(q2) + cos(q3) + 4, cos(q2 + q3)/2 + (3*cos(q2))/2 + cos(q3) + 5/3, cos(q2 + q3)/2 + cos(q3)/2 + 1/3;
cos(q2 + q3)/2 + (3*cos(q2))/2 + cos(q3) + 5/3,                                  cos(q3) + 5/3,                  cos(q3)/2 + 1/3;
              cos(q2 + q3)/2 + cos(q3)/2 + 1/3,                                cos(q3)/2 + 1/3,                              1/3];

    assert(isequal(M, M'),'error')

== matlab function Lorenzo_comparison_simulation/Liu/MATLAB Function ==
  data: u_des input; M input; y input; y output; C input; u_sc input; norm_u_tot output
function [y,norm_u_tot]= dynamics(u_des, M,y, C, u_sc)
    
    q = reshape(y(1:3),[3,1]);
    dq = reshape(y(4:6),[3,1]);



    [~, p] = chol(M);
    decision = (p == 0);

    assert(decision, 'Inertia matrix is not positive definite');
    
    u_tot = u_des + u_sc;
    norm_u_tot=norm(u_tot);
    ddq = inv(M) * (u_tot - C * dq ); 

    y = [dq; ddq];

== matlab function Lorenzo_comparison_simulation/Liu/MATLAB Function2 ==
  data: y input; C output
function C = coriolis(y)

    q1 = y(1);
    q2 = y(2);
    q3 = y(3);
    dq1 = y(4);
    dq2 = y(5);
    dq3 = y(6);


    C = [- dq2*(sin(q2 + q3)/2 + (3*sin(q2))/2) - dq3*(sin(q2 + q3)/2 + sin(q3)/2), - dq1*(sin(q2 + q3)/2 + (3*sin(q2))/2) - dq2*(sin(q2 + q3)/2 + (3*sin(q2))/2) - dq3*(sin(q2 + q3)/2 + sin(q3)/2), - dq1*(sin(q2 + q3)/2 + sin(q3)/2) - dq2*(sin(q2 + q3)/2 + sin(q3)/2) - dq3*(sin(q2 + q3)/2 + sin(q3)/2);
                dq1*(sin(q2 + q3)/2 + (3*sin(q2))/2) - (dq3*sin(q3))/2,                                                                                                 -(dq3*sin(q3))/2,                                                    - (dq1*sin(q3))/2 - (dq2*sin(q3))/2 - (dq3*sin(q3))/2;
                       dq1*(sin(q2 + q3)/2 + sin(q3)/2) + (dq2*sin(q3))/2,                                                                                (dq1*sin(q3))/2 + (dq2*sin(q3))/2,                                                                                                        0];

== matlab function Lorenzo_comparison_simulation/Liu/MATLAB Function3 ==
  data: C input; y input; cbf_control output; M input; h input; dh_dq input; hessian input; u_des input; psi_nominal output; psi_safety output; computed_H_dot output; cbf output; cbf_dot_nominal output; cbf_dot_safety output; alpha input; gamma input; damp input

function [cbf_control, psi_nominal, psi_safety, computed_H_dot, cbf, cbf_dot_nominal,cbf_dot_safety]= CBF(C, y, M, h, dh_dq, hessian, u_des, alpha, gamma, damp)
    
    q = reshape(y(1:3),[3,1]);
    dq = reshape(y(4:6),[3,1]);
    dh_dq = reshape(dh_dq,[1,3]);

    M_inv = inv(M);

    cbf =  h + alpha * dh_dq * dq;

    cbf_dot_nominal =  dh_dq * dq + alpha * dq' * hessian * dq + alpha * dh_dq * (M_inv* (-C * dq + u_des));
    psi_nominal = cbf_dot_nominal + gamma .* cbf;
    if psi_nominal<0
        lg_h = alpha * dh_dq * M_inv;
        cbf_control =  - lg_h' /(lg_h * lg_h')  .* psi_nominal;
    else
        cbf_control = zeros(3,1);
    end
    cbf_dot_safety = dh_dq * dq + alpha * dq' * hessian * dq + alpha * dh_dq * (M_inv* (-C * dq + u_des + cbf_control));
    psi_safety = cbf_dot_safety + gamma .* cbf;

    computed_H_dot = dq' * cbf_control - dq' * damp * dq;
    
end



% 
% function [cbf_control, psi_nominal, psi_safety, computed_H_dot, cbf, cbf_dot_nominal,cbf_dot_safety]= CBF(y, M, h, dh_dq, alpha, damp)
% 
%     q = reshape(y(1:2),[2,1]);
%     dq = reshape(y(3:4),[2,1]);
%     dh_dq = reshape(dh_dq,[1,2]);
% 
% 
%     KE = 0.5 * dq' * M * dq;
%     cbf = 1/h + KE/(1+KE);
%     lg_h = dq'/(1+KE)^2;
%     cbf_dot_nominal = - 1/h^2 * (dh_dq * dq)- 1/(1+KE)^2 * dq' * damp * dq;
%     psi_nominal = cbf_dot_nominal - alpha .* h;
%     if psi_nominal>0
% 
%         cbf_control =  -lg_h' /(lg_h*lg_h')  .* psi_nominal;
%     else
%         cbf_control = zeros(2,1);
%     end
%     cbf_dot_safety =  - 1/h^2 * (dh_dq * dq)- 1/(1+KE)^2 * dq' * damp * dq + lg_h * cbf_control;
%     psi_safety = cbf_dot_safety - alpha .* h;
% 
%     computed_H_dot = dq' * cbf_control - dq' * damp * dq;
% 
% end

== matlab function Lorenzo_comparison_simulation/Liu/MATLAB Function4 ==
  data: y input; h output; dh_dq output; hessian_sym output; geometry input
function [h, dh_dq, hessian_sym] = obstacle(y, geometry)
    % Define numerical values for the parameters
    % xc = 2.5;
    % yc = 2;
    % r = 1;

    xc = geometry(1);
    yc = geometry(2);
    r = geometry(3);

    l1 = 1;
    l2 = 1;
    l3 = 1;
    
    % Compute the end-effector position using forward kinematics
    q1 = y(1);
    q2 = y(2);
    q3 = y(3);
    
    x_ee = l1 * cos(q1) + l2 * cos(q1 + q2) + l3 * cos(q1 + q2 + q3);
    y_ee = l1 * sin(q1) + l2 * sin(q1 + q2) + l3 * sin(q1 + q2 + q3);
    
    % Compute the control barrier function h
    h = (xc - x_ee)^2 + (yc - y_ee)^2 - r^2;
    
    % Define the expressions for dh_dq and hessian_sym
    dh_dq = [2*(cos(q1 + q2 + q3) + cos(q1 + q2) + cos(q1))*(sin(q1 + q2 + q3) + sin(q1 + q2) + sin(q1) - 2) - 2*(sin(q1 + q2 + q3) + sin(q1 + q2) + sin(q1))*(cos(q1 + q2 + q3) + cos(q1 + q2) + cos(q1) - 5/2), 2*(cos(q1 + q2 + q3) + cos(q1 + q2))*(sin(q1 + q2 + q3) + sin(q1 + q2) + sin(q1) - 2) - 2*(sin(q1 + q2 + q3) + sin(q1 + q2))*(cos(q1 + q2 + q3) + cos(q1 + q2) + cos(q1) - 5/2), 2*cos(q1 + q2 + q3)*(sin(q1 + q2 + q3) + sin(q1 + q2) + sin(q1) - 2) - 2*sin(q1 + q2 + q3)*(cos(q1 + q2 + q3) + cos(q1 + q2) + cos(q1) - 5/2)];


    hessian_sym = [                                              2*(cos(q1 + q2 + q3) + cos(q1 + q2) + cos(q1))^2 - 2*(cos(q1 + q2 + q3) + cos(q1 + q2) + cos(q1))*(cos(q1 + q2 + q3) + cos(q1 + q2) + cos(q1) - 5/2) + 2*(sin(q1 + q2 + q3) + sin(q1 + q2) + sin(q1))^2 - 2*(sin(q1 + q2 + q3) + sin(q1 + q2) + sin(q1))*(sin(q1 + q2 + q3) + sin(q1 + q2) + sin(q1) - 2), 2*(cos(q1 + q2 + q3) + cos(q1 + q2))*(cos(q1 + q2 + q3) + cos(q1 + q2) + cos(q1)) - 2*(cos(q1 + q2 + q3) + cos(q1 + q2))*(cos(q1 + q2 + q3) + cos(q1 + q2) + cos(q1) - 5/2) + 2*(sin(q1 + q2 + q3) + sin(q1 + q2))*(sin(q1 + q2 + q3) + sin(q1 + q2) + sin(q1)) - 2*(sin(q1 + q2 + q3) + sin(q1 + q2))*(sin(q1 + q2 + q3) + sin(q1 + q2) + sin(q1) - 2), 2*cos(q1 + q2 + q3)*(cos(q1 + q2 + q3) + cos(q1 + q2) + cos(q1)) - 2*cos(q1 + q2 + q3)*(cos(q1 + q2 + q3) + cos(q1 + q2) + cos(q1) - 5/2) + 2*sin(q1 + q2 + q3)*(sin(q1 + q2 + q3) + sin(q1 + q2) + sin(q1)) - 2*sin(q1 + q2 + q3)*(sin(q1 + q2 + q3) + sin(q1 + q2) + sin(q1) - 2);
        2*(cos(q1 + q2 + q3) + cos(q1 + q2))*(cos(q1 + q2 + q3) + cos(q1 + q2) + cos(q1)) - 2*(cos(q1 + q2 + q3) + cos(q1 + q2))*(cos(q1 + q2 + q3) + cos(q1 + q2) + cos(q1) - 5/2) + 2*(sin(q1 + q2 + q3) + sin(q1 + q2))*(sin(q1 + q2 + q3) + sin(q1 + q2) + sin(q1)) - 2*(sin(q1 + q2 + q3) + sin(q1 + q2))*(sin(q1 + q2 + q3) + sin(q1 + q2) + sin(q1) - 2),                                                                                       2*(cos(q1 + q2 + q3) + cos(q1 + q2))^2 - 2*(cos(q1 + q2 + q3) + cos(q1 + q2))*(cos(q1 + q2 + q3) + cos(q1 + q2) + cos(q1) - 5/2) + 2*(sin(q1 + q2 + q3) + sin(q1 + q2))^2 - 2*(sin(q1 + q2 + q3) + sin(q1 + q2))*(sin(q1 + q2 + q3) + sin(q1 + q2) + sin(q1) - 2),                     2*cos(q1 + q2 + q3)*(cos(q1 + q2 + q3) + cos(q1 + q2)) - 2*cos(q1 + q2 + q3)*(cos(q1 + q2 + q3) + cos(q1 + q2) + cos(q1) - 5/2) - 2*sin(q1 + q2 + q3)*(sin(q1 + q2 + q3) + sin(q1 + q2) + sin(q1) - 2) + 2*sin(q1 + q2 + q3)*(sin(q1 + q2 + q3) + sin(q1 + q2));
                                                                            2*cos(q1 + q2 + q3)*(cos(q1 + q2 + q3) + cos(q1 + q2) + cos(q1)) - 2*cos(q1 + q2 + q3)*(cos(q1 + q2 + q3) + cos(q1 + q2) + cos(q1) - 5/2) + 2*sin(q1 + q2 + q3)*(sin(q1 + q2 + q3) + sin(q1 + q2) + sin(q1)) - 2*sin(q1 + q2 + q3)*(sin(q1 + q2 + q3) + sin(q1 + q2) + sin(q1) - 2),                                                                                         2*cos(q1 + q2 + q3)*(cos(q1 + q2 + q3) + cos(q1 + q2)) - 2*cos(q1 + q2 + q3)*(cos(q1 + q2 + q3) + cos(q1 + q2) + cos(q1) - 5/2) - 2*sin(q1 + q2 + q3)*(sin(q1 + q2 + q3) + sin(q1 + q2) + sin(q1) - 2) + 2*sin(q1 + q2 + q3)*(sin(q1 + q2 + q3) + sin(q1 + q2)),                                                                                       2*cos(q1 + q2 + q3)^2 - 2*cos(q1 + q2 + q3)*(cos(q1 + q2 + q3) + cos(q1 + q2) + cos(q1) - 5/2) + 2*sin(q1 + q2 + q3)^2 - 2*sin(q1 + q2 + q3)*(sin(q1 + q2 + q3) + sin(q1 + q2) + sin(q1) - 2)];
     

    % d = eig(hessian_sym)
    % isposdef = all(d >= 0);
    % 
    % assert(isposdef, 'error hessian');
end

== matlab function Lorenzo_comparison_simulation/Liu/MATLAB Function5 ==
  data: spring input; damp input; y input; out output; q_d input
function out  = u_des( spring, damp, y, q_d)


    q = reshape(y(1:3),[3,1]);
    dq = reshape(y(4:6),[3,1]);


    
    out =  - damp * dq - spring * (q-q_d);

== matlab function Lorenzo_comparison_simulation/Liu/MATLAB Function6 ==
  data: M input; E output; y input; spring input; q_d input; T output; V output
function [E,T,V] = energy(M,y,spring, q_d)
    q = y(1:3);
    dq = y(4:6);
    
    T = 0.5 * (dq' * M * dq) ;
    V =0.5 * spring *(q-q_d)' * (q-q_d);
    E = T + V;
